simulink model "Sim_System_Param_Estimator_2022b"  (R2022b)
settings: Solver=FixedStepAuto  StartTime=0.0  StopTime=20  FixedStep=0.05  RelTol=1e-3
undefined symbols (not defined in the file or in its folder): A, B
settings Model: Creator=RAOUF  LastModifiedBy=Claudia Yasar
settings DataIOCC: ReturnWorkspaceOutputs=off
settings OptimizationCC: ReuseModelBlockBuffer=on

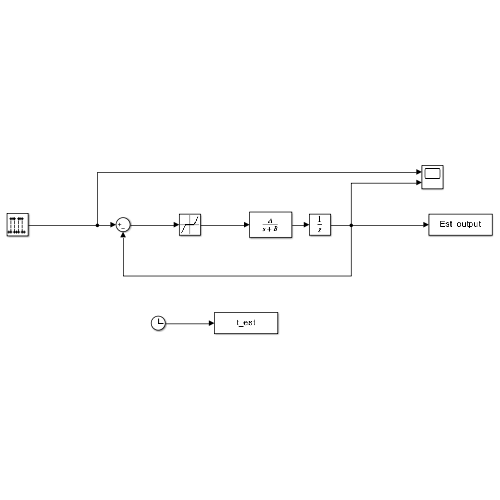
[thumbnail: Simulink's stored preview of the top-level diagram]
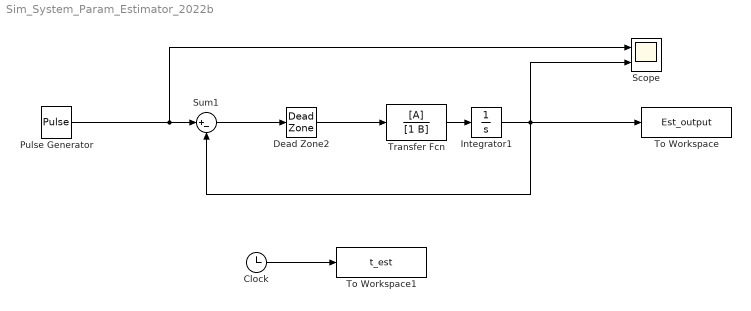
== system Sim_System_Param_Estimator_2022b ==
  Clock : Clock
  Dead Zone2 : DeadZone  LowerValue=-0.05  UpperValue=0.05
  Integrator1 : Integrator
  Pulse Generator : DiscretePulseGenerator  Amplitude=pi/3  Period=40  PulseWidth=20  PhaseDelay=5  SampleTime=0.05
  Scope : Scope  NumInputPorts=2
  Sum1 : Sum  Inputs=|+-
  To Workspace : ToWorkspace  VariableName=Est_output  SampleTime=-1
      settings: Save2DSignal=2-D array (concatenate along first dimension)
  To Workspace1 : ToWorkspace  VariableName=t_est  SampleTime=-1
      settings: Save2DSignal=2-D array (concatenate along first dimension)
  Transfer Fcn : TransferFcn  Numerator=[A]  Denominator=[1 B]
  wires:
  Transfer Fcn/1 -> Integrator1/1
  Dead Zone2/1 -> Transfer Fcn/1
  Sum1/1 -> Dead Zone2/1
  Pulse Generator/1 -> Scope/1, Sum1/1
  Integrator1/1 -> To Workspace/1, Sum1/2, Scope/2
  Clock/1 -> To Workspace1/1
